simulink model "control_dig_"  (R2017b)
settings: Solver=VariableStepAuto  StartTime=0.0  StopTime=10  RelTol=1e-3
values from neighbouring files (symbols this model uses):
  gcd = c2d(gc,Tm,'tustin')    [control_digital.m]
  gcda = c2d(g_ca,Tm)    [control_digital.m]
  Kp = 4.48    [control_digital.m]
  p0 = x(4)    [control_algebraico_dig.m]    (also in control_digital.m = 583)
  p1 = x(3)    [control_algebraico_dig.m]    (also in control_digital.m = 39)
  p2 = 1    [control_digital.m]
  q0 = x(2)    [control_algebraico_dig.m]    (also in control_digital.m = 200)
  q1 = x(1)    [control_algebraico_dig.m]    (also in control_digital.m = 526.64)
  q2 = 151.8    [control_digital.m]
  Td = 0.1741    [control_digital.m]
  Ti = 2.24    [control_digital.m]
  Tm = 0.01    [control_algebraico_dig.m]    (also in control_digital.m)
libraries: simulink x3
settings Model: Creator=Acer  LastModifiedBy=franj
settings DataIOCC: ReturnWorkspaceOutputs=on
settings SFSimCC: SimUseLocalCustomCode=on
settings RTWCC: RTWUseLocalCustomCode=on

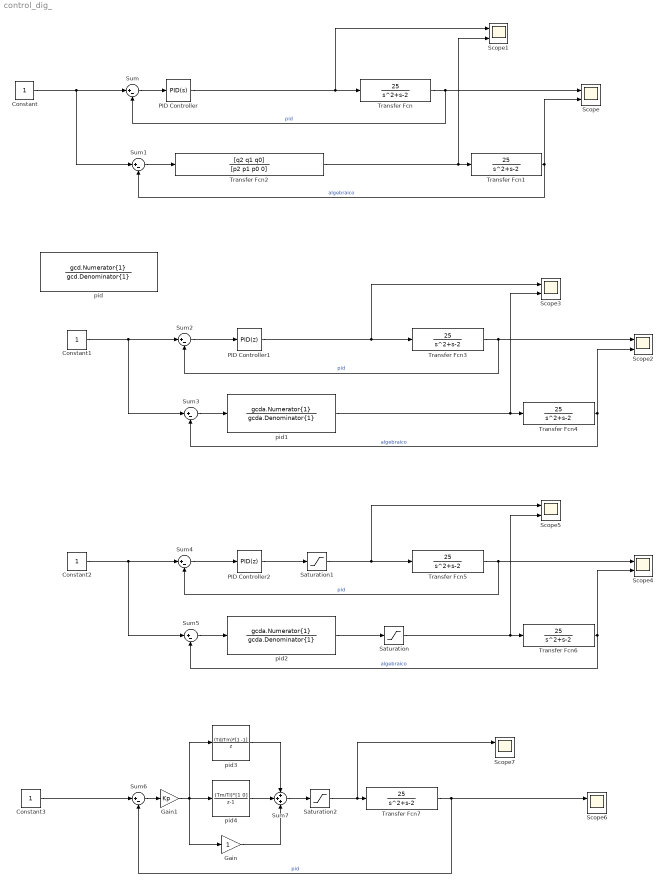
== system control_dig_ ==
  Constant{,1..3} (4 alike) : Constant
  Gain : Gain
  Gain1 : Gain  Gain=Kp
  PID Controller : simulink/Continuous/PID Controller  Controller=PID  Form=Parallel  TimeDomain=Continuous-time  SampleTime=-1  IntegratorMethod=Forward Euler  FilterMethod=Forward Euler  ControllerParametersSource=internal  P=Kp  I=Kp/Ti  D=Kp*Td  UseFilter=on  N=100  TunerSelectOption=Transfer Function Based (PID Tuner App)  InitialConditionSource=internal  InitialConditionForIntegrator=0  InitialConditionForFilter=0  DifferentiatorICPrevScaledInput=0  ExternalReset=none  TrackingMode=off  Kt=1  LimitOutput=off  UpperSaturationLimit=inf  LowerSaturationLimit=-inf  LinearizeAsGain=on  AntiWindupMode=none  Kb=1  POutMin=[]  POutMax=[]  IOutMin=[]  IOutMax=[]  DOutMin=[]  DOutMax=[]  NOutMin=[]  NOutMax=[]  SumOutMin=[]  SumOutMax=[]  SaturationOutMin=[]  SaturationOutMax=[]  PParamMin=[]  PParamMax=[]  IParamMin=[]  IParamMax=[]  DParamMin=[]  DParamMax=[]  NParamMin=[]  NParamMax=[]  KbParamMin=[]  KbParamMax=[]  KtParamMin=[]  KtParamMax=[]  KbOutMin=[]  KbOutMax=[]  KtOutMin=[]  KtOutMax=[]  IntegratorOutMin=[]  IntegratorOutMax=[]  FilterOutMin=[]  FilterOutMax=[]  SumI1OutMin=[]  SumI1OutMax=[]  SumI2OutMin=[]  SumI2OutMax=[]  SumI3OutMin=[]  SumI3OutMax=[]  SumDOutMin=[]  SumDOutMax=[]  DifferentiatorOutMin=[]  DifferentiatorOutMax=[]  FilterDiffOutCoefMin=[]  FilterDiffOutCoefMax=[]  ReciprocalOutMin=[]  ReciprocalOutMax=[]  SumDenOutMin=[]  SumDenOutMax=[]  SumNumOutMin=[]  SumNumOutMax=[]  DivideOutMin=[]  DivideOutMax=[]  IntegratorContinuousStateAttributes=''  IntegratorStateMustResolveToSignalObject=off  IntegratorRTWStateStorageClass=Auto  FilterContinuousStateAttributes=''  FilterStateMustResolveToSignalObject=off  FilterRTWStateStorageClass=Auto  InitialConditionSetting=State (most efficient)
  PID Controller1 : simulink/Continuous/PID Controller  Controller=PID  Form=Parallel  TimeDomain=Discrete-time  SampleTime=Tm  IntegratorMethod=Forward Euler  FilterMethod=Forward Euler  ControllerParametersSource=internal  P=Kp  I=(Kp/Ti)  D=Kp*Td  UseFilter=on  N=100  TunerSelectOption=Transfer Function Based (PID Tuner App)  InitialConditionSource=internal  InitialConditionForIntegrator=0  InitialConditionForFilter=0  DifferentiatorICPrevScaledInput=0  ExternalReset=none  TrackingMode=off  Kt=1  LimitOutput=off  UpperSaturationLimit=10  LowerSaturationLimit=-10  LinearizeAsGain=on  AntiWindupMode=none  Kb=1  POutMin=[]  POutMax=[]  IOutMin=[]  IOutMax=[]  DOutMin=[]  DOutMax=[]  NOutMin=[]  NOutMax=[]  SumOutMin=[]  SumOutMax=[]  SaturationOutMin=[]  SaturationOutMax=[]  PParamMin=[]  PParamMax=[]  IParamMin=[]  IParamMax=[]  DParamMin=[]  DParamMax=[]  NParamMin=[]  NParamMax=[]  KbParamMin=[]  KbParamMax=[]  KtParamMin=[]  KtParamMax=[]  KbOutMin=[]  KbOutMax=[]  KtOutMin=[]  KtOutMax=[]  IntegratorOutMin=[]  IntegratorOutMax=[]  FilterOutMin=[]  FilterOutMax=[]  SumI1OutMin=[]  SumI1OutMax=[]  SumI2OutMin=[]  SumI2OutMax=[]  SumI3OutMin=[]  SumI3OutMax=[]  SumDOutMin=[]  SumDOutMax=[]  DifferentiatorOutMin=[]  DifferentiatorOutMax=[]  FilterDiffOutCoefMin=[]  FilterDiffOutCoefMax=[]  ReciprocalOutMin=[]  ReciprocalOutMax=[]  SumDenOutMin=[]  SumDenOutMax=[]  SumNumOutMin=[]  SumNumOutMax=[]  DivideOutMin=[]  DivideOutMax=[]  IntegratorContinuousStateAttributes=''  IntegratorStateMustResolveToSignalObject=off  IntegratorRTWStateStorageClass=Auto  FilterContinuousStateAttributes=''  FilterStateMustResolveToSignalObject=off  FilterRTWStateStorageClass=Auto  InitialConditionSetting=State (most efficient)
  PID Controller2 : simulink/Continuous/PID Controller  Controller=PID  Form=Parallel  TimeDomain=Discrete-time  SampleTime=Tm  IntegratorMethod=Forward Euler  FilterMethod=Forward Euler  ControllerParametersSource=internal  P=Kp  I=(Kp/Ti)  D=Kp*Td  UseFilter=on  N=100  TunerSelectOption=Transfer Function Based (PID Tuner App)  InitialConditionSource=internal  InitialConditionForIntegrator=0  InitialConditionForFilter=0  DifferentiatorICPrevScaledInput=0  ExternalReset=none  TrackingMode=off  Kt=1  LimitOutput=off  UpperSaturationLimit=10  LowerSaturationLimit=-10  LinearizeAsGain=on  AntiWindupMode=none  Kb=1  POutMin=[]  POutMax=[]  IOutMin=[]  IOutMax=[]  DOutMin=[]  DOutMax=[]  NOutMin=[]  NOutMax=[]  SumOutMin=[]  SumOutMax=[]  SaturationOutMin=[]  SaturationOutMax=[]  PParamMin=[]  PParamMax=[]  IParamMin=[]  IParamMax=[]  DParamMin=[]  DParamMax=[]  NParamMin=[]  NParamMax=[]  KbParamMin=[]  KbParamMax=[]  KtParamMin=[]  KtParamMax=[]  KbOutMin=[]  KbOutMax=[]  KtOutMin=[]  KtOutMax=[]  IntegratorOutMin=[]  IntegratorOutMax=[]  FilterOutMin=[]  FilterOutMax=[]  SumI1OutMin=[]  SumI1OutMax=[]  SumI2OutMin=[]  SumI2OutMax=[]  SumI3OutMin=[]  SumI3OutMax=[]  SumDOutMin=[]  SumDOutMax=[]  DifferentiatorOutMin=[]  DifferentiatorOutMax=[]  FilterDiffOutCoefMin=[]  FilterDiffOutCoefMax=[]  ReciprocalOutMin=[]  ReciprocalOutMax=[]  SumDenOutMin=[]  SumDenOutMax=[]  SumNumOutMin=[]  SumNumOutMax=[]  DivideOutMin=[]  DivideOutMax=[]  IntegratorContinuousStateAttributes=''  IntegratorStateMustResolveToSignalObject=off  IntegratorRTWStateStorageClass=Auto  FilterContinuousStateAttributes=''  FilterStateMustResolveToSignalObject=off  FilterRTWStateStorageClass=Auto  InitialConditionSetting=State (most efficient)
  Saturation : Saturate  UpperLimit=10  LowerLimit=-10
  Saturation1 : Saturate  UpperLimit=10  LowerLimit=-10
  Saturation2 : Saturate  UpperLimit=10  LowerLimit=-10
  Scope{,1..7} (8 alike) : Scope  NumInputPorts=2
  Sum{,1..6} (7 alike) : Sum  Inputs=|+-
  Sum7 : Sum  Inputs=+++
  Transfer Fcn{,1,3..7} (7 alike) : TransferFcn  Numerator=[25]  Denominator=[1 1 -2]
  Transfer Fcn2 : TransferFcn  Numerator=[q2 q1 q0]  Denominator=[p2 p1 p0 0]
  pid : DiscreteTransferFcn  Numerator=gcd.Numerator{1}  Denominator=gcd.Denominator{1}  SampleTime=Tm
  pid1 : DiscreteTransferFcn  Numerator=gcda.Numerator{1}  Denominator=gcda.Denominator{1}  SampleTime=Tm
  pid2 : DiscreteTransferFcn  Numerator=gcda.Numerator{1}  Denominator=gcda.Denominator{1}  SampleTime=Tm
  pid3 : DiscreteTransferFcn  Numerator=(Td/Tm)*[1 -1]  Denominator=[1 0]  SampleTime=Tm
  pid4 : DiscreteTransferFcn  Numerator=(Tm/Ti)*[1 0]  Denominator=[1 -1]  SampleTime=Tm
  wires:
  Sum/1 -> PID Controller/1
  PID Controller/1 -> Scope1/1, Transfer Fcn/1
  Transfer Fcn/1 -> Scope/1, Sum/2  "pid"
  Sum1/1 -> Transfer Fcn2/1
  Transfer Fcn2/1 -> Scope1/2, Transfer Fcn1/1
  Transfer Fcn1/1 -> Scope/2, Sum1/2  "algebraico"
  Constant/1 -> Sum1/1, Sum/1
  Constant1/1 -> Sum3/1, Sum2/1
  Sum2/1 -> PID Controller1/1
  PID Controller1/1 -> Scope3/1, Transfer Fcn3/1
  Sum3/1 -> pid1/1
  Transfer Fcn3/1 -> Scope2/1, Sum2/2  "pid"
  Transfer Fcn4/1 -> Scope2/2, Sum3/2  "algebraico"
  pid1/1 -> Scope3/2, Transfer Fcn4/1
  PID Controller2/1 -> Saturation1/1
  Sum4/1 -> PID Controller2/1
  Transfer Fcn6/1 -> Scope4/2, Sum5/2  "algebraico"
  pid2/1 -> Saturation/1
  Transfer Fcn5/1 -> Scope4/1, Sum4/2  "pid"
  Constant2/1 -> Sum5/1, Sum4/1
  Sum5/1 -> pid2/1
  Saturation1/1 -> Scope5/1, Transfer Fcn5/1
  Saturation/1 -> Scope5/2, Transfer Fcn6/1
  Saturation2/1 -> Scope7/1, Transfer Fcn7/1
  Constant3/1 -> Sum6/1
  Transfer Fcn7/1 -> Scope6/1, Sum6/2  "pid"
  Sum7/1 -> Saturation2/1
  Sum6/1 -> Gain1/1
  pid3/1 -> Sum7/1
  pid4/1 -> Sum7/2
  Gain/1 -> Sum7/3
  Gain1/1 -> Gain/1, pid3/1, pid4/1
